simulink model "Simulink_Model"  (R2018b)
settings: Solver=FixedStepAuto  StartTime=0.0  StopTime=T_sim  FixedStep=SAMPLE_TIME  RelTol=1e-12
values from neighbouring files (symbols this model uses):
  CONTROLLER_INITIAL_CONDITION = 0    [Parameter.m]
  CONVERSION_COSTANT_1 = 0.341159914008612    (= 0.341159914009)    [Parameter.m]
  CONVERSION_COSTANT_2 = 0.000416568624689888    (= 0.00041656862469)    [Parameter.m]
  Final_Step_Value = input("Final Step Value [bar]: ")    [Parameter.m]
  Initial_Step_Value = input("Initial Step Value [bar]: ")    [Parameter.m]
  k_i = 0    [Parameter.m]
  k_p = 3    [Parameter.m]
  MODEL_INITIAL_CONDITION = 0    [Parameter.m]
  OUTPUT_WHEN_ON = 78    [Parameter.m]
  Step_Time = T_sim/2    [Parameter.m]
  SWITCH_POINT = 1    [Parameter.m]
  Time_Delay = input("Feedback delay [s]: ")    [Parameter.m]
settings Model: Creator=paoloesposito  LastModifiedBy=Alessandro
settings SolverCC: ZeroCrossAlgorithm=Adaptive
settings DebuggingCC: MaxConsecutiveZCsMsg=none  LibraryContextMissingDiagnostic=none
settings SFSimCC: SimUseLocalCustomCode=off
settings RTWCC: RTWUseLocalCustomCode=off

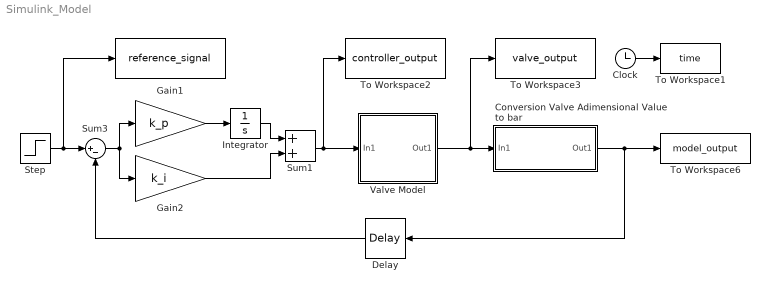
== system Simulink_Model ==
  " " : ToWorkspace  VariableName=reference_signal  SampleTime=-1
  Clock : Clock
  "Conversion Valve Adimensional Value to bar " : Subsystem
  Delay : TransportDelay  DelayTime=Time_Delay  BufferSize=21504
  Gain1 : Gain  Gain=k_p
  Gain2 : Gain  Gain=k_i
  Integrator : Integrator  InitialCondition=CONTROLLER_INITIAL_CONDITION
  Step : Step  Time=Step_Time  Before=Initial_Step_Value  After=Final_Step_Value  SampleTime=0
  Sum1 : Sum
  Sum3 : Sum  Inputs=|+-
  To Workspace1 : ToWorkspace  VariableName=time  SampleTime=-1
  To Workspace2 : ToWorkspace  VariableName=controller_output  SampleTime=-1
  To Workspace3 : ToWorkspace  VariableName=valve_output  SampleTime=-1
  To Workspace6 : ToWorkspace  VariableName=model_output  SampleTime=-1
  Valve Model : Subsystem
  wires:
  Clock/1 -> To Workspace1/1
  Gain1/1 -> Integrator/1
  Delay/1 -> Sum3/2
  Sum3/1 -> Gain2/1, Gain1/1
  Step/1 -> " "/1, Sum3/1
  "Conversion Valve Adimensional Value to bar "/1(Out1) -> To Workspace6/1, Delay/1
  Valve Model/1(Out1) -> To Workspace3/1, "Conversion Valve Adimensional Value to bar "/1(In1)
  Sum1/1 -> To Workspace2/1, Valve Model/1(In1)
  Integrator/1 -> Sum1/1
  Gain2/1 -> Sum1/2

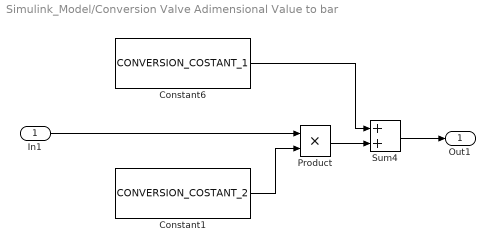
== system Simulink_Model/Conversion Valve Adimensional Value to bar  ==
  In1 : Inport
  Constant1 : Constant  Value=CONVERSION_COSTANT_2
  Constant6 : Constant  Value=CONVERSION_COSTANT_1
  Product : Product
  Sum4 : Sum
  Out1 : Outport
  wires:
  Constant6/1 -> Sum4/1
  Sum4/1 -> Out1/1
  In1/1 -> Product/1
  Product/1 -> Sum4/2
  Constant1/1 -> Product/2

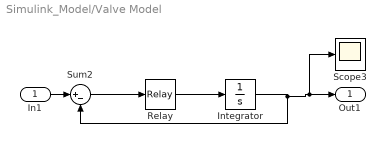
== system Simulink_Model/Valve Model ==
  In1 : Inport
  Integrator : Integrator  InitialCondition=MODEL_INITIAL_CONDITION
  Relay : Relay  OnSwitchValue=SWITCH_POINT  OffSwitchValue=-SWITCH_POINT  OnOutputValue=OUTPUT_WHEN_ON  OffOutputValue=-OUTPUT_WHEN_ON
  Scope3 : Scope
  Sum2 : Sum  Inputs=|+-
  Out1 : Outport
  wires:
  In1/1 -> Sum2/1
  Relay/1 -> Integrator/1
  Integrator/1 -> Scope3/1, Out1/1, Sum2/2
  Sum2/1 -> Relay/1
